simulink library "MultiUser_Lib"  (R2018b)
settings: Solver=VariableStepAuto  StartTime=0.0  StopTime=10.0  RelTol=1e-3
settings Model: Creator=HP  LastModifiedBy=Victor.Oke
settings SFSimCC: SimUseLocalCustomCode=off
settings RTWCC: RTWUseLocalCustomCode=off
settings CodeAppCC: StateflowObjectComments=on

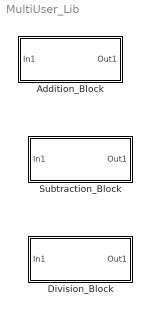
== system MultiUser_Lib ==
  Addition_Block : Subsystem
  Division_Block : Subsystem
  Subtraction_Block : Subsystem

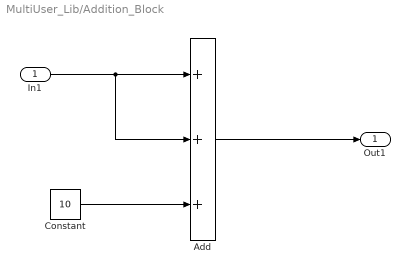
== system MultiUser_Lib/Addition_Block ==
  In1 : Inport
  Add : Sum  Inputs=+++
  Constant : Constant  Value=10  OutDataTypeStr=double
  Out1 : Outport
  wires:
  In1/1 -> Add/2, Add/1
  Add/1 -> Out1/1
  Constant/1 -> Add/3

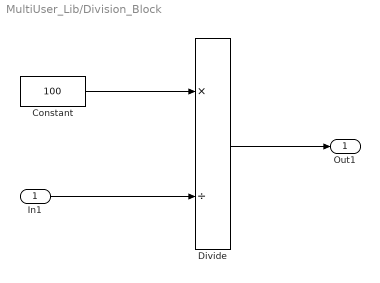
== system MultiUser_Lib/Division_Block ==
  In1 : Inport
  Constant : Constant  Value=100  OutDataTypeStr=double
  Divide : Product  Inputs=*/
  Out1 : Outport
  wires:
  In1/1 -> Divide/2
  Constant/1 -> Divide/1
  Divide/1 -> Out1/1

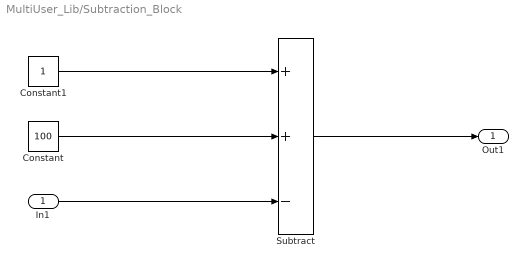
== system MultiUser_Lib/Subtraction_Block ==
  In1 : Inport
  Constant : Constant  Value=100  OutDataTypeStr=double
  Constant1 : Constant
  Subtract : Sum  Inputs=++-
  Out1 : Outport
  wires:
  Subtract/1 -> Out1/1
  In1/1 -> Subtract/3
  Constant/1 -> Subtract/2
  Constant1/1 -> Subtract/1
